simulink library "navlib1"  (Simulink 2.09)
undefined symbols (not defined in the file or in its folder): Sgs, Sloc
libraries: navlib1 x5

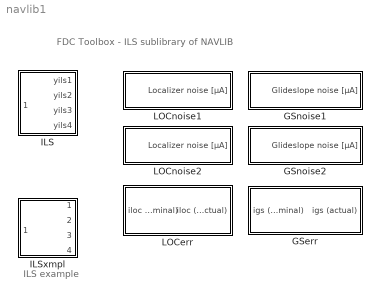
== system navlib1 ==
  note: ILS example
  note: FDC Toolbox - ILS sublibrary of NAVLIB
  GSerr : Subsystem  mask(GS steady-state errors){cat=2}
      mask prompts: cat "Performance category (1, 2, or 3):"
      mask help: Glideslope steady-state errors
      mask init:
      | gamgs=-abs(@4*pi/180); Sgs=625/abs(gamgs); if cat == 1, D_igs=Sgs*0.075*gamgs; KSgs=1+(@2/100)*0.25; elseif cat == 2, D_igs=Sgs*0.075*gamgs;  KSgs=1+(@2/100)*0.20; else, D_igs=Sgs*0.04*gamgs; KSgs=1+(@2/100)*0.15; end; D_igs=D_igs*@3/100;
      mask Help: eval('fdchelp gserr')
      mask Display: disp('Glideslope steady\nstate errors\nAGARD R-632')
  GSnoise1 : Subsystem  mask(GsNoise1){Lgs=85, sigma_gs=15, V=40}
      mask prompts: Lgs "Scale length Lgs [m]:"; sigma_gs "Standard deviation sigma_gs [µA]:"; V "Approach speed [m/s]:"
      mask help: Glideslope noise (AGARD R-632)
      mask init:
      | K=sigma_gs*sqrt(2*Lgs/V); tau=Lgs/V;
      mask Help: eval('fdchelp gsnoise')
      mask Display: disp('GS noise\nAGARD R-632')
  GSnoise2 : Subsystem
      mask Type: GSNoise NASA-CR2022
      mask Description:
      | Glideslope Noise
      | (NASA-CR2022)
      mask Help: eval('fdchelp gsnoise')
      mask Display: disp('GS noise\nNASA CR-2022')
  ILS : Subsystem  mask(ILS){RWpos=[20000,-100,0]}
      mask prompts: RWpos "Heading of runway [deg]:"
      mask help: Approach: ILS
      mask init:
      | psiRW=@1*pi/180; cos_psiRW=cos(psiRW); sin_psiRW=sin(psiRW); xloc=abs(@3); xgs=abs(@4); ygs=-abs(@5); gamgs=-abs(@6)*pi/180; tan_gamgs=tan(gamgs); cos_gamgs=cos(gamgs); Sgs=625/abs(gamgs); if xloc == 0, Sloc = 1; else, Sloc=1.4*xloc; end;
      mask Help: eval('fdchelp ils')
      mask Display: disp('Nominal\nILS\nsignals')
  ILSxmpl : Subsystem
      mask Display: plot(0,0,100,100,[53,23,30,61,53],[45,60,64,49,45],[16,27,32,26],[48,40,43,47],[21,20,24,26,21],[44,55,56,47,44],[20,20,16],[50,50,48],[38,27,26,33],[52,46,48,55],[42,38,27],[50,47,46],[40,44,44,45,45,44,42],[48,44,42,42,44,44,50],[47,45,43],[55,58,58],[54,84,98,90,54],[36,21,56,58,36],[74,68],[34,29],[81,76],[43,38],[87,83],[49,45],[94,89],[57,52],[105,105],[0,0])
  LOCerr : Subsystem  mask(LOC steady-state errors){cat=2, xloc=2200}
      mask prompts: cat "Performance category (1, 2, or 3):"; xloc "% of max. allowable error in localizer sensitivity:"
      mask help: Localizer steady-state errors
      mask init:
      | Sloc = 1.4*xloc; if cat == 1, D_iloc=Sloc*atan(10.5/xloc); KSloc=1+(@2/100)*0.17; elseif cat == 2, D_iloc=Sloc*atan(7.5/xloc);  KSloc=1+(@2/100)*0.17; else, D_iloc=Sloc*atan(3/xloc); KSloc=1+(@2/100)*0.10; end; D_iloc=D_iloc*@3/100;
      mask Help: eval('fdchelp locerr')
      mask Display: disp('Localizer steady\nstate errors\nAGARD R-632')
  LOCnoise1 : Subsystem  mask(LocNoise1){Lloc=130, sigma_loc=15, V=40}
      mask prompts: Lloc "Scale length Lloc [m]:"; sigma_loc "Standard deviation sigma_loc [µA]:"; V "Approach speed [m/s]:"
      mask help: Localizer noise (AGARD R-632)
      mask init:
      | K=sigma_loc*sqrt(2*Lloc/V); tau=Lloc/V;
      mask Help: eval('fdchelp locnoise')
      mask Display: disp('LOC noise\nAGARD R-632')
  LOCnoise2 : Subsystem
      mask Type: LocNoise 2
      mask Description:
      | Localizer noise
      | (NASA-CR2022)
      mask Help: eval('fdchelp locnoise')
      mask Display: disp('LOC noise\nNASA CR-2022')

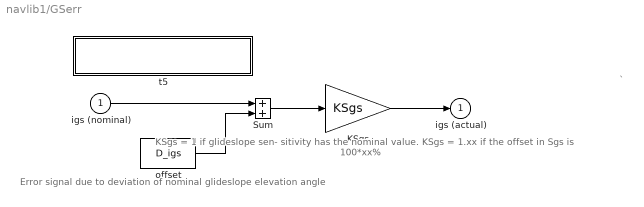
== system navlib1/GSerr ==
  note: `
  note: Error signal due to deviation
      | of nominal glideslope
      | elevation angle
  note: KSgs = 1 if glideslope sen-
      | sitivity has the nominal value.
      | KSgs = 1.xx if the offset in
      | Sgs is 100*xx%
  igs (nominal) : Inport  Port=1  PortWidth=-1  SampleTime=-1
  KSgs : Gain  Gain=KSgs
  Sum : Sum  Inputs=++
  offset : Constant  Value=D_igs
  t5 : Subsystem
      settings: OpenFcn=fdchelp gserr
      mask Display: disp('Glideslope steady-state errors\nMarc Rauw, October 1997')
  igs (actual) : Outport  Port=1  InitialOutput=0
  wires:
  KSgs/1 -> igs (actual)/1
  Sum/1 -> KSgs/1
  igs (nominal)/1 -> Sum/1
  offset/1 -> Sum/2

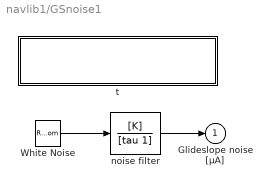
== system navlib1/GSnoise1 ==
  White Noise : RandomNumber  Mean=0  Variance=1  Seed=200  SampleTime=-1
  noise filter : TransferFcn  Numerator=[K]  Denominator=[tau 1]
  t : Subsystem
      settings: OpenFcn=fdchelp gsnoise
      mask Display: disp('Glideslope noise AGARD R-632\n(constant approach speed)\nMarc Rauw, October 1997')
  Glideslope noise [µA] : Outport  Port=1  InitialOutput=0
  wires:
  White Noise/1 -> noise filter/1
  noise filter/1 -> Glideslope noise [µA]/1

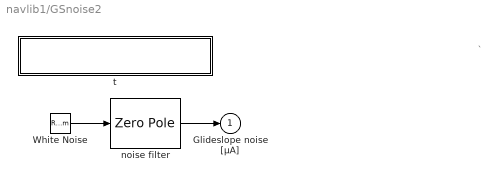
== system navlib1/GSnoise2 ==
  note: `
  White Noise : RandomNumber  Mean=0  Variance=1  Seed=200  SampleTime=-1
  noise filter : ZeroPole  Zeros=[]  Poles=[-0.25]  Gain=[3.9875]
  t : Subsystem
      settings: OpenFcn=fdchelp gsnoise
      mask Display: disp('Glideslope noise NASA CR2022\nMarc Rauw, October 1997')
  Glideslope noise [µA] : Outport  Port=1  InitialOutput=0
  wires:
  noise filter/1 -> Glideslope noise [µA]/1
  White Noise/1 -> noise filter/1

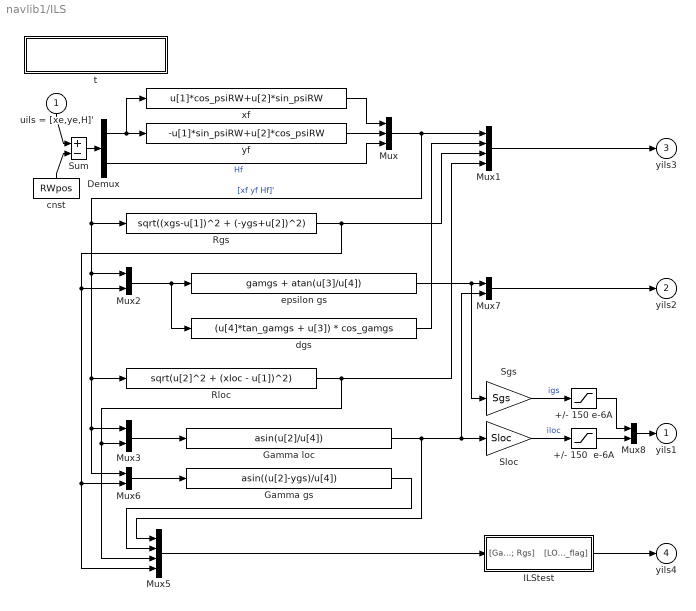
== system navlib1/ILS ==
  uils = [xe,ye,H]' : Inport  Orientation=down  Port=1  PortWidth=-1  SampleTime=-1
  +/- 150  e-6A : Saturate  UpperLimit=150  LowerLimit=-150
  +/- 150 e-6A : Saturate  UpperLimit=150  LowerLimit=-150
  Demux : Demux  Outputs=[2 1]
  Gamma gs : Fcn  Expr=asin((u[2]-ygs)/u[4])
  Gamma loc : Fcn  Expr=asin(u[2]/u[4])
  ILStest : Subsystem
      mask Type: ILStest
      mask Description: ILS coverage test
      mask Help: eval('fdchelp ilstest')
      mask Display: disp('ILS coverage\ntest (LOC & GS)')
  Mux : Mux  Inputs=3
  Mux1 : Mux  Inputs=[3 1 1 1]
  Mux2 : Mux  Inputs=[3 1]
  Mux3 : Mux  Inputs=[3 1]
  Mux5 : Mux  Inputs=4
  Mux6 : Mux  Inputs=[3 1]
  Mux7 : Mux  Inputs=2
  Mux8 : Mux  Inputs=2
  Rgs : Fcn  Expr=sqrt((xgs-u[1])^2 + (-ygs+u[2])^2)
  Rloc : Fcn  Expr=sqrt(u[2]^2 + (xloc - u[1])^2)
  Sgs : Gain  Gain=Sgs
  Sloc : Gain  Gain=Sloc
  Sum : Sum  Inputs=+-
  cnst : Constant  Orientation=up  Value=RWpos
  dgs : Fcn  Expr=(u[4]*tan_gamgs + u[3]) * cos_gamgs
  epsilon gs : Fcn  Expr=gamgs + atan(u[3]/u[4])
  t : Subsystem
      settings: OpenFcn=fdchelp ils
      mask Display: disp('Nominal ILS signals\nM.O. Rauw, January 1998')
  xf : Fcn  Expr=u[1]*cos_psiRW+u[2]*sin_psiRW
  yf : Fcn  Expr=-u[1]*sin_psiRW+u[2]*cos_psiRW
  yils1 : Outport  Port=1  InitialOutput=0
  yils2 : Outport  Port=2  InitialOutput=0
  yils3 : Outport  Port=3  InitialOutput=0
  yils4 : Outport  Port=4  InitialOutput=0
  wires:
  Gamma gs/1 -> Mux5/2
  Mux5/1 -> ILStest/1("[Gamma_loc; Gamma_gs; Rloc; Rgs]")
  ILStest/1("[LOC_flag; GS_flag]") -> yils4/1
  Gamma loc/1 -> Mux5/1, Sloc/1, Mux7/2
  Mux6/1 -> Gamma gs/1
  Mux2/1 -> epsilon gs/1, dgs/1
  Mux1/1 -> yils3/1
  Rloc/1 -> Mux1/4, Mux3/2, Mux5/3
  dgs/1 -> Mux1/2
  Mux3/1 -> Gamma loc/1
  yf/1 -> Mux/2
  xf/1 -> Mux/1
  Sgs/1 -> +/- 150 e-6A/1  "igs"
  Sloc/1 -> +/- 150  e-6A/1  "iloc"
  +/- 150  e-6A/1 -> Mux8/2
  Mux7/1 -> yils2/1
  +/- 150 e-6A/1 -> Mux8/1
  Mux8/1 -> yils1/1
  Rgs/1 -> Mux1/3, Mux2/2, Mux6/2, Mux5/4
  uils = [xe,ye,H]'/1 -> Sum/1
  cnst/1 -> Sum/2
  Demux/2 -> Mux/3  "Hf"
  epsilon gs/1 -> Mux7/1, Sgs/1
  Mux/1 -> Mux2/1, Rloc/1, Mux3/1, Mux6/1, Rgs/1, Mux1/1  "[xf yf Hf]'"
  Sum/1 -> Demux/1
  Demux/1 -> yf/1, xf/1

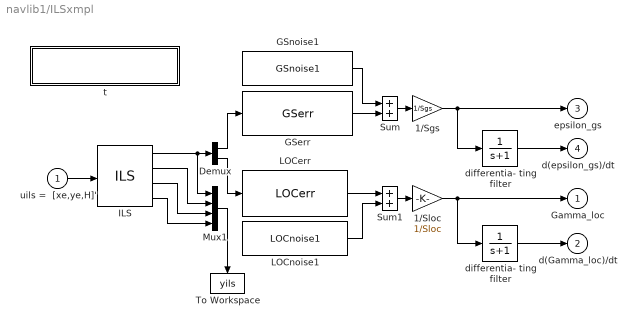
== system navlib1/ILSxmpl ==
  uils =  [xe,ye,H]' : Inport  Port=1  PortWidth=-1  SampleTime=-1
  1/Sgs : Gain  Gain=1/Sgs
  1/Sloc : Gain  Gain=1/Sloc
  Demux : Demux  Outputs=2
  GSerr : navlib1/GSerr  cat=2  MaskParam2=100  MaskParam3=100  MaskParam4=-3
  GSnoise1 : navlib1/GSnoise1  Lgs=85  sigma_gs=15  V=40
  ILS : navlib1/ILS  RWpos=[20000,-100,0]  MaskParam1=0  MaskParam3=2200  MaskParam4=300  MaskParam5=100  MaskParam6=3
  LOCerr : navlib1/LOCerr  cat=2  xloc=2200  MaskParam2=100  MaskParam3=100
  LOCnoise1 : navlib1/LOCnoise1  Lloc=130  sigma_loc=15  V=40
  Mux1 : Mux  Inputs=[2 2 6 2]
  Sum : Sum  Inputs=++
  Sum1 : Sum  Inputs=++
  To Workspace : ToWorkspace  VariableName=yils  SampleTime=0
      settings: Orientation=down  Buffer=5000
  differentia- ting filter : TransferFcn  Numerator=[1]  Denominator=[1 1]
  "differentia- ting filter " : TransferFcn  Numerator=[1]  Denominator=[1 1]
  t : Subsystem
      settings: OpenFcn=fdchelp ilsxmpl
      mask Display: disp('ILS example\nMarc Rauw, April 1998')
  Gamma_loc : Outport  Port=1  InitialOutput=0
  d(Gamma_loc)/dt : Outport  Port=2  InitialOutput=0
  epsilon_gs : Outport  Port=3  InitialOutput=0
  d(epsilon_gs)/dt : Outport  Port=4  InitialOutput=0
  wires:
  1/Sgs/1 -> epsilon_gs/1, "differentia- ting filter "/1
  "differentia- ting filter "/1 -> d(epsilon_gs)/dt/1
  1/Sloc/1 -> Gamma_loc/1, differentia- ting filter/1
  differentia- ting filter/1 -> d(Gamma_loc)/dt/1
  Mux1/1 -> To Workspace/1
  Demux/1 -> GSerr/1
  Demux/2 -> LOCerr/1
  GSerr/1 -> Sum/2
  LOCnoise1/1 -> Sum1/2
  uils =  [xe,ye,H]'/1 -> ILS/1
  Sum/1 -> 1/Sgs/1
  Sum1/1 -> 1/Sloc/1
  ILS/4 -> Mux1/4
  ILS/1 -> Demux/1, Mux1/1
  ILS/3 -> Mux1/3
  GSnoise1/1 -> Sum/1
  ILS/2 -> Mux1/2
  LOCerr/1 -> Sum1/1

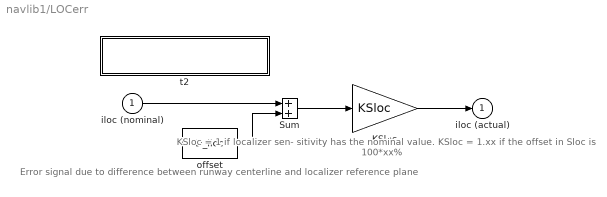
== system navlib1/LOCerr ==
  note: Error signal due to difference
      | between runway centerline and
      | localizer reference plane
  note: KSloc = 1 if localizer sen-
      | sitivity has the nominal value.
      | KSloc = 1.xx if the offset in
      | Sloc is 100*xx%
  iloc (nominal) : Inport  Port=1  PortWidth=-1  SampleTime=-1
  KSloc : Gain  Gain=KSloc
  Sum : Sum  Inputs=++
  offset : Constant  Value=D_iloc
  t2 : Subsystem
      settings: OpenFcn=fdchelp locerr
      mask Display: disp('Localizer steady-state errors\nMarc Rauw, October 1997')
  iloc (actual) : Outport  Port=1  InitialOutput=0
  wires:
  offset/1 -> Sum/2
  iloc (nominal)/1 -> Sum/1
  Sum/1 -> KSloc/1
  KSloc/1 -> iloc (actual)/1

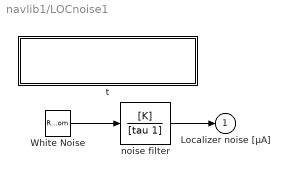
== system navlib1/LOCnoise1 ==
  White Noise : RandomNumber  Mean=0  Variance=1  Seed=100  SampleTime=-1
  noise filter : TransferFcn  Numerator=[K]  Denominator=[tau 1]
  t : Subsystem
      settings: OpenFcn=fdchelp locnoise
      mask Display: disp('Localizer noise AGARD R-632\n(constant approach speed)\nMarc Rauw, October 1997')
  Localizer noise [µA] : Outport  Port=1  InitialOutput=0
  wires:
  noise filter/1 -> Localizer noise [µA]/1
  White Noise/1 -> noise filter/1

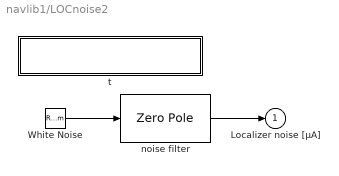
== system navlib1/LOCnoise2 ==
  White Noise : RandomNumber  Mean=0  Variance=1  Seed=100  SampleTime=-1
  noise filter : ZeroPole  Zeros=[-1.5]  Poles=[-0.35; -10]  Gain=[5]
  t : Subsystem
      settings: OpenFcn=fdchelp locnoise
      mask Display: disp('Localizer noise NASA CR2022\nMarc Rauw, October 1997')
  Localizer noise [µA] : Outport  Port=1  InitialOutput=0
  wires:
  White Noise/1 -> noise filter/1
  noise filter/1 -> Localizer noise [µA]/1

== system navlib1/GSerr/t5 ==
  note: T

== system navlib1/GSnoise1/t ==
  note: T

== system navlib1/GSnoise2/t ==

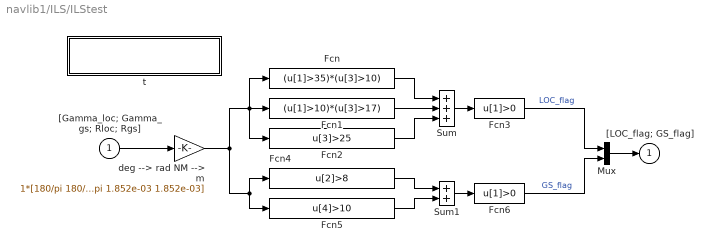
== system navlib1/ILS/ILStest ==
  "[Gamma_loc; Gamma_gs; Rloc; Rgs]" : Inport  Port=1  PortWidth=-1  SampleTime=-1
  Fcn : Fcn  Expr=(u[1]>35)*(u[3]>10)
  Fcn1 : Fcn  Expr=(u[1]>10)*(u[3]>17)
  Fcn2 : Fcn  Expr=u[3]>25
  Fcn3 : Fcn  Expr=u[1]>0
  Fcn4 : Fcn  Expr=u[2]>8
  Fcn5 : Fcn  Expr=u[4]>10
  Fcn6 : Fcn  Expr=u[1]>0
  Mux : Mux  Inputs=2
  Sum : Sum  Inputs=+++
  Sum1 : Sum  Inputs=++
  deg --> rad NM --> m : Gain  Gain=1*[180/pi 180/pi 1.852e-03 1.852e-03]
  t : Subsystem
      settings: OpenFcn=fdchelp ilstest
      mask Display: disp('ILStest (coverage test)\nM.O. Rauw, October 1997')
  "[LOC_flag; GS_flag]" : Outport  Port=1  InitialOutput=0
  wires:
  "[Gamma_loc; Gamma_gs; Rloc; Rgs]"/1 -> deg --> rad NM --> m/1
  Sum1/1 -> Fcn6/1
  Fcn5/1 -> Sum1/2
  Fcn4/1 -> Sum1/1
  Sum/1 -> Fcn3/1
  Fcn2/1 -> Sum/3
  Fcn1/1 -> Sum/2
  Fcn/1 -> Sum/1
  Mux/1 -> "[LOC_flag; GS_flag]"/1
  Fcn3/1 -> Mux/1  "LOC_flag"
  Fcn6/1 -> Mux/2  "GS_flag"
  deg --> rad NM --> m/1 -> Fcn4/1, Fcn5/1, Fcn1/1, Fcn/1, Fcn2/1

== system navlib1/ILS/t ==

== system navlib1/ILSxmpl/t ==

== system navlib1/LOCerr/t2 ==
  note: T

== system navlib1/LOCnoise1/t ==

== system navlib1/LOCnoise2/t ==

== system navlib1/ILS/ILStest/t ==
